simulink model "PV_MG_DroopMPPTV4_TwoFarms"  (R2015a)
settings: Solver=ode3  StartTime=0.0  StopTime=inf  FixedStep=5e-5  RelTol=1e-3
undefined symbols (not defined in the file): Ion, Lithium
libraries: powerlib x61, powerlib_meascontrol x12, simulink x10, fuzblock x3, simulink_extras x3, re_lib x2, electricdrivelib x1
(part 1 of 2)
settings Model: PauseTimes=1.45  CovModelRefEnable=off  Creator=Nady  LastModifiedBy=Nady
settings DataIOCC: SaveFormat=StructureWithTime
settings HardwareCC: ProdBitPerPointer=64  ProdLargestAtomicFloat=Float  ProdIntDivRoundTo=Zero  ProdEndianess=LittleEndian  ProdHWDeviceType=Specified
settings GRTTargetCC: GeneratePreprocessorConditionals=Use local settings

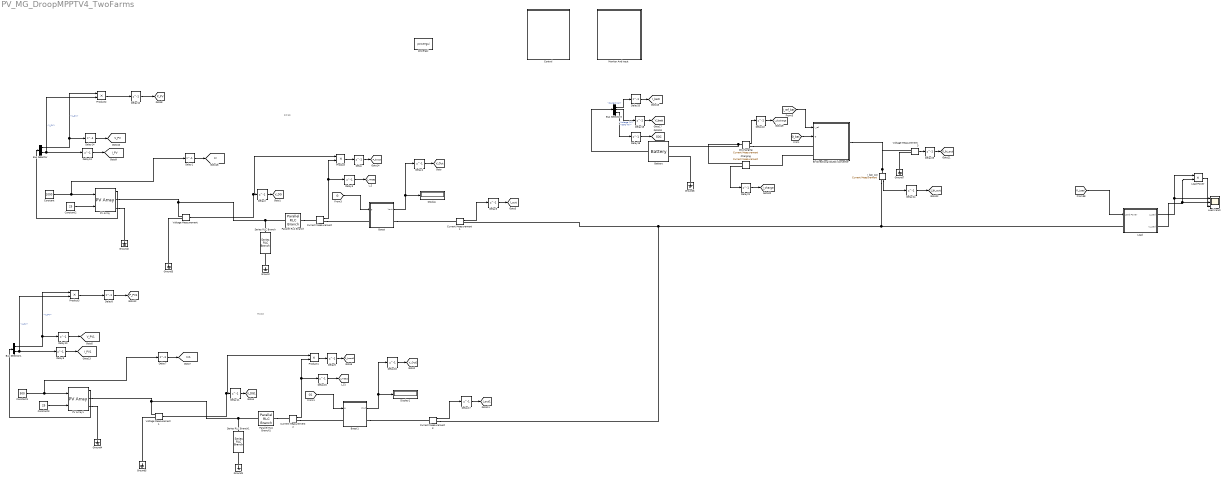
== system PV_MG_DroopMPPTV4_TwoFarms ==
  note: R=10
  note: R=10
  Battery : electricdrivelib/Extra Sources/Battery  BatType=Lithium-Ion  ShowTempParam=off  ThermalPreset=no  NomV=30  NomQ=5.4  SOC=100  Batt_Tr=15  PresetModel=on  MaxQ=5.4  FullV=34.9196  Dis_rate=2.3478  R=0.055556  Normal_OP=4.8835  expZone="[32.4116     0.265304]"  current=[6.5 13 32.5]  Units=Time  Tci=20  NomT=20  T2=-30  MaxQ2=4.8  FullV2=7.1  Normal_OP2=5.72  expZone2="[6.58  1]"  Rca=0.6  ti=1000
  Bi-Directional DC/DC Converter : Subsystem
  Boost : Subsystem
  Boost1 : Subsystem
  Bus Selector : BusSelector  OutputSignals=V_PV,I_PV
  Bus Selector1 : BusSelector  OutputSignals=V_PV,I_PV
  Bus Selector3 : BusSelector  OutputSignals=Current (A),Voltage (V),SOC (%)
  Charging : powerlib/Measurements/Current Measurement  PhasorSimulation=off  OutputType=Complex  PSBequivalent=0
  Constant : Constant  Value=1000
  Constant1 : Constant  Value=500
  Constant2 : Constant  Value=25
  Constant3 : Constant  Value=25
  "Control " : Subsystem
  Current Measurement{,1..3} (4 alike) : powerlib/Measurements/Current Measurement  PhasorSimulation=off  OutputType=Complex  PSBequivalent=0
  Delay{,1..24} (25 alike) : Delay  DelayLength=1  InitialCondition=0
  Discharging : powerlib/Measurements/Current Measurement  PhasorSimulation=off  OutputType=Complex  PSBequivalent=0
  Display : Display
  Display1 : Display
  Ground{,1..7} (8 alike) : powerlib/Elements/Ground  LConnTagsString=a
  I_bat_out : powerlib/Measurements/Current Measurement  PhasorSimulation=off  OutputType=Complex  PSBequivalent=0
  Load : Subsystem
  Load Power : Product
  Load Vand I : Scope  NumInputPorts=3
      settings: TimeRange=auto  MaxDataPoints=5000  SaveToWorkspace=off  SaveName=ScopeData2  YMin=-350.25555~2.15805~-1449.82848  YMax=3150.38643~330.92882~4956.57534  SampleTime=-1
  Monitor And Input : Subsystem
  PV Array : re_lib/Solar/PV Array  Npar=5  Nser=1  PlotType=one module @ 25 deg.C & specified irradiances  S_vec="[ 1000  800 ]"  Temp_C_vec=[35]  ModuleName=Sun Earth Solar Power TDB125x125-36-P 80W  PlotWhenSelected=off  Pm=80.004  Ncell=36  Voc=21.9  Isc=5  Vm=17.7  Im=4.52  beta_Voc_pc=-0.32  alpha_Isc_pc=0.04  beta_Voc=-0.07008  alpha_Isc=0.002  IL=5.0238  I0=3.6974e-11  nI=0.92596  Rsh=70.2892  Rs=0.35567  BAL=off  Tc=1e-6  Tfilter=5e-5
  PV Array1 : re_lib/Solar/PV Array  Npar=5  Nser=1  PlotType=one module @ 25 deg.C & specified irradiances  S_vec="[ 1000  800 ]"  Temp_C_vec=[35]  ModuleName=Sun Earth Solar Power TDB125x125-36-P 80W  PlotWhenSelected=off  Pm=80.004  Ncell=36  Voc=21.9  Isc=5  Vm=17.7  Im=4.52  beta_Voc_pc=-0.32  alpha_Isc_pc=0.04  beta_Voc=-0.07008  alpha_Isc=0.002  IL=5.0238  I0=3.6974e-11  nI=0.92596  Rsh=70.2892  Rs=0.35567  BAL=off  Tc=1e-6  Tfilter=5e-5
  Parallel RLC Branch : powerlib/Elements/Parallel RLC Branch  LConnTagsString=a  RConnTagsString=__new0  BranchType=RL  Resistance=10  Inductance=0.0164  SetiL0=off  InitialCurrent=0  Capacitance=1e-6  Setx0=off  InitialVoltage=0  Measurements=None
  Parallel RLC Branch1 : powerlib/Elements/Parallel RLC Branch  LConnTagsString=a  RConnTagsString=__new0  BranchType=RL  Resistance=10  Inductance=0.0164  SetiL0=off  InitialCurrent=0  Capacitance=1e-6  Setx0=off  InitialVoltage=0  Measurements=None
  Product{,1..3} (4 alike) : Product
  Series RLC Branch : powerlib/Elements/Series RLC Branch  LConnTagsString=__new0  RConnTagsString=__new0  BranchType=C  Resistance=0.1  Inductance=1e-3  SetiL0=off  InitialCurrent=0  Capacitance=0.1  Setx0=off  InitialVoltage=0  Measurements=None
  Series RLC Branch1 : powerlib/Elements/Series RLC Branch  LConnTagsString=__new0  RConnTagsString=__new0  BranchType=C  Resistance=0.1  Inductance=1e-3  SetiL0=off  InitialCurrent=0  Capacitance=0.1  Setx0=off  InitialVoltage=0  Measurements=None
  Voltage Measurement : powerlib/Measurements/Voltage Measurement  PhasorSimulation=off  OutputType=Complex  PSBequivalent=0
  Voltage Measurement1 : powerlib/Measurements/Voltage Measurement  PhasorSimulation=off  OutputType=Complex  PSBequivalent=0
  Voltage Measurement3 : powerlib/Measurements/Voltage Measurement  PhasorSimulation=off  OutputType=Complex  PSBequivalent=0
  powergui : powerlib/powergui  Priority=1  SimulationMode=Discrete  SolverType=Tustin  SampleTime=5e-5  frequency=60  SPID=off  DisableSnubberDevices=off  DisableRonSwitches=off  DisableVfSwitches=off  SwTol=0  DisplayEquations=off  Interpol=off  ExternalGateDelay=off  methode=on  Ts=20  FunctionMessages=off  echomessages=off  HookPort=off  EnableUseOfTLC=off  x0status=blocks  frequencyindice=0  Pbase=100e6  ErrMax=1e-4  Iterations=50  UnitsV=kV  UnitsW=MW  buscounter=0  RestoreLinks=warning  ResistiveCurrentMeasurement=off  Frange=[0:2:500]  Ylog=off  Xlog=on  ShowGrid=off  save=off  variable=ZData  structure=0  ZoomFFT=off  StartTime=0.0  cycles=1  DisplayStyle=1  fundamental=60  FreqAxis=off  MaxFrequency=1000  frequencyindicesteady=1  RmsSteady=1  display=off
  tag scope: I_PV1=global, I_PV=global, I_batt=global, I_bi_out=global, I_charge=global, I_discharge=global, I_meas1=global, I_meas=global, I_out1=global, I_out=global, Irr1=global, Irr=global, P_PV1=global, P_PV=global, P_boost1=global, P_boost=global, SOC=global, V_DG1=global, V_DG=global, V_Out1=global, V_Out=global, V_PV1=global, V_PV=global, V_batt=global, V_bi_out=global
  wires:
  Boost/1(Vout) -> Display/1, Delay4/1
  Voltage Measurement/1 -> Delay2/1, Product/1
  Current Measurement/1 -> Product/2, Delay3/1
  [P_Load] -> Load/1(Load Power)
  Load/1(I_Load) -> Load Power/1, Load Vand I/1
  Load/2(V_Load) -> Load Power/2, Load Vand I/2
  Load Power/1 -> Load Vand I/3
  Current Measurement1/1 -> Delay5/1
  Product/1 -> Delay/1
  Delay/1 -> [P_boost]
  Delay1/1 -> [Irr]
  Delay2/1 -> [V_DG]
  Delay3/1 -> [I_meas]
  Delay4/1 -> [V_Out]
  Delay5/1 -> [I_out]
  Constant2/1 -> PV Array/2
  Bus Selector/1 -> Delay14/1, Product2/1  "<V_PV>"
  Bus Selector/2 -> Delay13/1, Product2/2  "<I_PV>"
  PV Array/1 -> Bus Selector/1
  Constant/1 -> PV Array/1, Delay1/1
  Product2/1 -> Delay12/1
  Delay12/1 -> [P_PV]
  [G] -> Boost/1(g)
  Delay13/1 -> [I_PV]
  Delay14/1 -> [V_PV]
  Boost1/1(Vout) -> Delay16/1, Display1/1
  Voltage Measurement1/1 -> Product1/1, Delay11/1
  Current Measurement2/1 -> Delay15/1, Product1/2
  Current Measurement3/1 -> Delay17/1
  Product1/1 -> Delay6/1
  Delay6/1 -> [P_boost1]
  Delay7/1 -> [Irr1]
  Delay11/1 -> [V_DG1]
  Delay15/1 -> [I_meas1]
  Delay16/1 -> [V_Out1]
  Delay17/1 -> [I_out1]
  Constant3/1 -> PV Array1/2
  Bus Selector1/1 -> Product3/1, Delay10/1  "<V_PV>"
  Bus Selector1/2 -> Product3/2, Delay9/1  "<I_PV>"
  PV Array1/1 -> Bus Selector1/1
  Constant1/1 -> Delay7/1, PV Array1/1
  Product3/1 -> Delay8/1
  Delay8/1 -> [P_PV1]
  [G1] -> Boost1/1(g)
  Delay9/1 -> [I_PV1]
  Delay10/1 -> [V_PV1]
  Discharging/1 -> Delay22/1
  Charging/1 -> Delay21/1
  [G_bat] -> Bi-Directional DC/DC Converter/2(G)
  Voltage Measurement3/1 -> Delay23/1
  I_bat_out/1 -> Delay24/1
  Battery/1 -> Bus Selector3/1
  Bus Selector3/1 -> Delay20/1  "<Current (A)>"
  Bus Selector3/2 -> Delay18/1  "<Voltage (V)>"
  [I_ref_bat] -> Bi-Directional DC/DC Converter/1(I_ref)
  Bus Selector3/3 -> Delay19/1  "<SOC (%)>"
  Delay19/1 -> [SOC]
  Delay18/1 -> [V_batt]
  Delay20/1 -> [I_batt]
  Delay21/1 -> [I_charge]
  Delay22/1 -> [I_discharge]
  Delay24/1 -> [I_bi_out]
  Delay23/1 -> [V_bi_out]
  connections:
  Current Measurement/RConn1 -- Boost/LConn1
  Voltage Measurement/LConn1 -- PV Array/RConn1 -- Parallel RLC Branch/LConn1 -- Series RLC Branch/LConn1
  Boost/RConn1 -- Current Measurement1/LConn1
  Load/LConn1 -- I_bat_out/RConn1 -- Current Measurement3/RConn1 -- Current Measurement1/RConn1
  Ground/LConn1 -- Series RLC Branch/RConn1
  PV Array/RConn2 -- Ground2/LConn1
  Voltage Measurement/LConn2 -- Ground3/LConn1
  Parallel RLC Branch/RConn1 -- Current Measurement/LConn1
  PV Array1/RConn1 -- Series RLC Branch1/LConn1 -- Parallel RLC Branch1/LConn1 -- Voltage Measurement1/LConn1
  Parallel RLC Branch1/RConn1 -- Current Measurement2/LConn1
  PV Array1/RConn2 -- Ground4/LConn1
  Voltage Measurement1/LConn2 -- Ground5/LConn1
  Current Measurement2/RConn1 -- Boost1/LConn1
  Ground1/LConn1 -- Series RLC Branch1/RConn1
  Boost1/RConn1 -- Current Measurement3/LConn1
  I_bat_out/LConn1 -- Bi-Directional DC/DC Converter/RConn1 -- Voltage Measurement3/LConn1
  Discharging/LConn1 -- Battery/LConn1 -- Charging/RConn1
  Ground7/LConn1 -- Voltage Measurement3/LConn2
  Ground6/LConn1 -- Battery/LConn2
  Discharging/RConn1 -- Bi-Directional DC/DC Converter/LConn1
  Bi-Directional DC/DC Converter/LConn2 -- Charging/LConn1

== system PV_MG_DroopMPPTV4_TwoFarms/Bi-Directional DC//DC Converter ==
  I_ref : Inport
  G : Inport  Port=2
  Boost : Subsystem
  Buck : Subsystem
  Constant2 : Constant  Value=0
  Constant3 : Constant  Value=0
  G1 : InportShadow  Port=2
  I_ref1 : InportShadow
  Switch1 : Switch  Criteria=u2 > Threshold
  Switch2 : Switch  Criteria=u2 > Threshold
  Boost_In : PMIOPort  Port=1  Side=Left
  V_Bus : PMIOPort  Port=2  Side=Right
  Buck_out : PMIOPort  Port=3  Side=Left
  wires:
  I_ref/1 -> Switch2/2
  Switch1/1 -> Buck/1(G)
  G/1 -> Switch1/3
  Switch2/1 -> Boost/1(g)
  G1/1 -> Switch2/1
  Constant2/1 -> Switch1/1
  Constant3/1 -> Switch2/3
  I_ref1/1 -> Switch1/2
  connections:
  Buck_out/RConn1 -- Buck/LConn1
  Boost_In/RConn1 -- Boost/LConn1
  Boost/RConn1 -- Buck/RConn1 -- V_Bus/RConn1

== system PV_MG_DroopMPPTV4_TwoFarms/Boost ==
  g : Inport
  C_LP : powerlib/Elements/Series RLC Branch  LConnTagsString=__new0  RConnTagsString=__new0  BranchType=R  Resistance=1  Inductance=1e-3  SetiL0=off  InitialCurrent=0  Capacitance=0.004  Setx0=off  InitialVoltage=0  Measurements=None
  Data Type Conversion : DataTypeConversion  OutDataTypeStr=boolean
  Ground : powerlib/Elements/Ground  LConnTagsString=a
  IGBT : powerlib/Power Electronics/IGBT  Ron=0.001  Lon=0  Vf=1  Tf=1e-6  Tt=2e-6  IC=0  Rs=1e5  Cs=inf  Measurements=on
  IGBT1 : powerlib/Power Electronics/IGBT  Ron=0.001  Lon=0  Vf=1  Tf=1e-6  Tt=2e-6  IC=0  Rs=1e5  Cs=inf  Measurements=on
  L_LP : powerlib/Elements/Series RLC Branch  LConnTagsString=__new0  RConnTagsString=__new0  BranchType=L  Resistance=0.01  Inductance=0.0164  SetiL0=off  InitialCurrent=0  Capacitance=6e-2  Setx0=off  InitialVoltage=0  Measurements=None
  Logical Operator : Logic  Operator=NOT  AllPortsSameDT=off  OutDataTypeStr=boolean
  R_LP1 : powerlib/Elements/Series RLC Branch  LConnTagsString=__new0  RConnTagsString=__new0  BranchType=L  Resistance=0.01  Inductance=7e-3  SetiL0=off  InitialCurrent=0  Capacitance=6e-2  Setx0=off  InitialVoltage=0  Measurements=None
  Series RLC Branch3 : powerlib/Elements/Series RLC Branch  LConnTagsString=__new0  RConnTagsString=__new0  BranchType=C  Resistance=0.005  Inductance=1e-3  SetiL0=off  InitialCurrent=0  Capacitance=6e-3  Setx0=off  InitialVoltage=0  Measurements=None
  Voltage Measurement : powerlib/Measurements/Voltage Measurement  PhasorSimulation=off  OutputType=Complex  PSBequivalent=0
  Vin (Il) : PMIOPort  Tag=PMCPort  Port=1  Side=Left
  Vc : PMIOPort  Tag=PMCPort  Port=2  Side=Right
  Vout : Outport
  wires:
  Voltage Measurement/1 -> Vout/1
  g/1 -> Data Type Conversion/1, IGBT/1
  Data Type Conversion/1 -> Logical Operator/1
  Logical Operator/1 -> IGBT1/1
  connections:
  IGBT/RConn1 -- Ground/LConn1 -- Voltage Measurement/LConn2 -- Series RLC Branch3/RConn1
  IGBT1/LConn1 -- R_LP1/LConn1 -- IGBT/LConn1
  R_LP1/RConn1 -- Vin (Il)/RConn1
  Vc/RConn1 -- C_LP/LConn1 -- L_LP/LConn1 -- Voltage Measurement/LConn1
  Series RLC Branch3/LConn1 -- C_LP/RConn1 -- L_LP/RConn1 -- IGBT1/RConn1

== system PV_MG_DroopMPPTV4_TwoFarms/Boost1 ==
  g : Inport
  C_LP : powerlib/Elements/Series RLC Branch  LConnTagsString=__new0  RConnTagsString=__new0  BranchType=R  Resistance=1  Inductance=1e-3  SetiL0=off  InitialCurrent=0  Capacitance=0.004  Setx0=off  InitialVoltage=0  Measurements=None
  Data Type Conversion : DataTypeConversion  OutDataTypeStr=boolean
  Ground : powerlib/Elements/Ground  LConnTagsString=a
  IGBT : powerlib/Power Electronics/IGBT  Ron=0.001  Lon=0  Vf=1  Tf=1e-6  Tt=2e-6  IC=0  Rs=1e5  Cs=inf  Measurements=on
  IGBT1 : powerlib/Power Electronics/IGBT  Ron=0.001  Lon=0  Vf=1  Tf=1e-6  Tt=2e-6  IC=0  Rs=1e5  Cs=inf  Measurements=on
  L_LP : powerlib/Elements/Series RLC Branch  LConnTagsString=__new0  RConnTagsString=__new0  BranchType=L  Resistance=0.01  Inductance=0.0164  SetiL0=off  InitialCurrent=0  Capacitance=6e-2  Setx0=off  InitialVoltage=0  Measurements=None
  Logical Operator : Logic  Operator=NOT  AllPortsSameDT=off  OutDataTypeStr=boolean
  R_LP1 : powerlib/Elements/Series RLC Branch  LConnTagsString=__new0  RConnTagsString=__new0  BranchType=L  Resistance=0.01  Inductance=7e-3  SetiL0=off  InitialCurrent=0  Capacitance=6e-2  Setx0=off  InitialVoltage=0  Measurements=None
  Series RLC Branch3 : powerlib/Elements/Series RLC Branch  LConnTagsString=__new0  RConnTagsString=__new0  BranchType=C  Resistance=0.005  Inductance=1e-3  SetiL0=off  InitialCurrent=0  Capacitance=6e-3  Setx0=off  InitialVoltage=0  Measurements=None
  Voltage Measurement : powerlib/Measurements/Voltage Measurement  PhasorSimulation=off  OutputType=Complex  PSBequivalent=0
  Vin (Il) : PMIOPort  Tag=PMCPort  Port=1  Side=Left
  Vc : PMIOPort  Tag=PMCPort  Port=2  Side=Right
  Vout : Outport
  wires:
  Logical Operator/1 -> IGBT1/1
  Data Type Conversion/1 -> Logical Operator/1
  g/1 -> IGBT/1, Data Type Conversion/1
  Voltage Measurement/1 -> Vout/1
  connections:
  IGBT1/RConn1 -- Series RLC Branch3/LConn1 -- L_LP/RConn1 -- C_LP/RConn1
  Voltage Measurement/LConn1 -- C_LP/LConn1 -- L_LP/LConn1 -- Vc/RConn1
  R_LP1/RConn1 -- Vin (Il)/RConn1
  IGBT/LConn1 -- R_LP1/LConn1 -- IGBT1/LConn1
  Series RLC Branch3/RConn1 -- Voltage Measurement/LConn2 -- Ground/LConn1 -- IGBT/RConn1

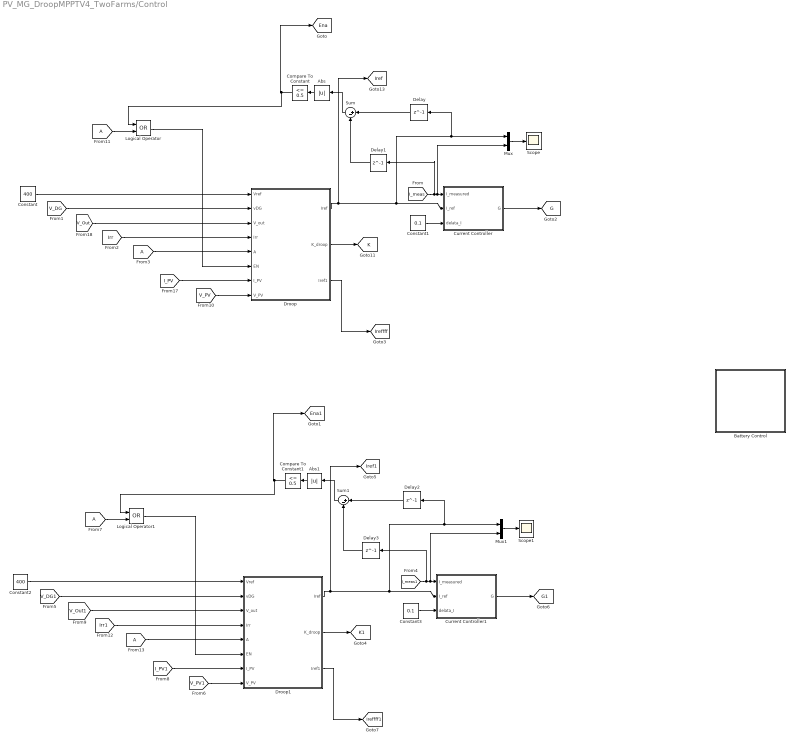
== system PV_MG_DroopMPPTV4_TwoFarms/Control  ==
  Abs : Abs
  Abs1 : Abs
  Battery Control : Subsystem
  Compare To Constant : simulink/Logic and Bit Operations/Compare To Constant  relop=<=  const=0.5  OutDataTypeStr=boolean
  Compare To Constant1 : simulink/Logic and Bit Operations/Compare To Constant  relop=<=  const=0.5  OutDataTypeStr=boolean
  Constant : Constant  Value=400  SampleTime=5e-5
  Constant1 : Constant  Value=0.1  SampleTime=0
  Constant2 : Constant  Value=400  SampleTime=5e-5
  Constant3 : Constant  Value=0.1  SampleTime=0
  Current Controller : Subsystem  TreatAsAtomicUnit=on
  Current Controller1 : Subsystem  TreatAsAtomicUnit=on
  Delay{,1..3} (4 alike) : Delay  DelayLength=1  InitialCondition=0
  Droop : Subsystem  TreatAsAtomicUnit=on
  Droop1 : Subsystem  TreatAsAtomicUnit=on
  Logical Operator : Logic  Operator=OR  AllPortsSameDT=off  OutDataTypeStr=boolean
  Logical Operator1 : Logic  Operator=OR  AllPortsSameDT=off  OutDataTypeStr=boolean
  Mux : Mux  Inputs=2
  Mux1 : Mux  Inputs=2
  Scope : Scope
      settings: TimeRange=auto  MaxDataPoints=5000  SaveToWorkspace=off  SaveName=ScopeData4  YMin=-2.92442  YMax=26.28218  SampleTime=-1
  Scope1 : Scope
      settings: TimeRange=auto  LimitDataPoints=on  MaxDataPoints=5000  SaveToWorkspace=off  YMin=-10  YMax=10  SampleTime=-1  DataFormat=Array
  Sum : Sum  Inputs=|+-
  Sum1 : Sum  Inputs=|+-
  tag scope: Ena1=global, Ena=global, G1=global, G=global, Iref1=global, Iref=global, Ireffff1=global, Ireffff=global, K1=global, K=global
  wires:
  Droop/1(Iref) -> Current Controller/2(I_ref), Delay/1, Mux/1, [Iref]
  Constant/1 -> Droop/1(Vref)
  [I_meas] -> Delay1/1, Mux/2, Current Controller/1(I_measured)
  Constant1/1 -> Current Controller/3(delata_I)
  Current Controller/1(G) -> [G]
  Droop/2(K_droop) -> [K]
  Mux/1 -> Scope/1
  Droop/3(Iref1) -> [Ireffff]
  Sum/1 -> Abs/1
  Abs/1 -> Compare To Constant/1
  Compare To Constant/1 -> Logical Operator/1, [Ena]
  Delay/1 -> Sum/1
  Delay1/1 -> Sum/2
  [V_DG] -> Droop/2(vDG)
  [V_Out] -> Droop/3(V_out)
  [Irr] -> Droop/4(Irr)
  [A] -> Droop/5(A)
  [I_PV] -> Droop/7(I_PV)
  [V_PV] -> Droop/8(V_PV)
  [A] -> Logical Operator/2
  Logical Operator/1 -> Droop/6(EN)
  Droop1/1(Iref) -> [Iref1], Mux1/1, Delay2/1, Current Controller1/2(I_ref)
  Constant2/1 -> Droop1/1(Vref)
  [I_meas1] -> Current Controller1/1(I_measured), Mux1/2, Delay3/1
  Constant3/1 -> Current Controller1/3(delata_I)
  Current Controller1/1(G) -> [G1]
  Droop1/2(K_droop) -> [K1]
  Mux1/1 -> Scope1/1
  Droop1/3(Iref1) -> [Ireffff1]
  Sum1/1 -> Abs1/1
  Abs1/1 -> Compare To Constant1/1
  Compare To Constant1/1 -> [Ena1], Logical Operator1/1
  Delay2/1 -> Sum1/1
  Delay3/1 -> Sum1/2
  [V_DG1] -> Droop1/2(vDG)
  [V_Out1] -> Droop1/3(V_out)
  [Irr1] -> Droop1/4(Irr)
  [A] -> Droop1/5(A)
  [I_PV1] -> Droop1/7(I_PV)
  [V_PV1] -> Droop1/8(V_PV)
  [A] -> Logical Operator1/2
  Logical Operator1/1 -> Droop1/6(EN)

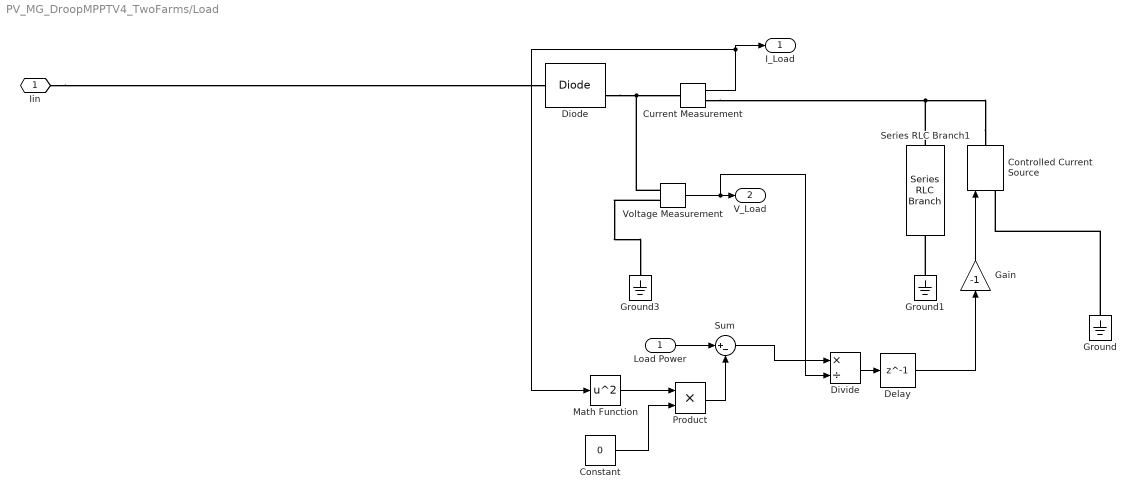
== system PV_MG_DroopMPPTV4_TwoFarms/Load ==
  Load Power : Inport
  Constant : Constant  Value=0
  Controlled Current Source : powerlib/Electrical Sources/Controlled Current Source  Initialize=on  Source_Type=AC  Amplitude=0  Phase=0  Frequency=0  Measurements=None
  Current Measurement : powerlib/Measurements/Current Measurement  PhasorSimulation=off  OutputType=Complex  PSBequivalent=0
  Delay : Delay  DelayLength=1  InitialCondition=0
  Diode : powerlib/Power Electronics/Diode  Ron=0.001  Lon=0  Vf=0.8  IC=0  UseSnubber=off  Rs=500  Cs=250e-9  Measurements=on
  Divide : Product  Inputs=*/
  Gain : Gain  Gain=-1
  Ground : powerlib/Elements/Ground  LConnTagsString=a
  Ground1 : powerlib/Elements/Ground  LConnTagsString=a
  Ground3 : powerlib/Elements/Ground  LConnTagsString=a
  Math Function : Math  Operator=square  SaturateOnIntegerOverflow=on
  Product : Product
  Series RLC Branch1 : powerlib/Elements/Series RLC Branch  LConnTagsString=__new0  RConnTagsString=__new0  BranchType=C  Resistance=1  Inductance=1e-3  SetiL0=off  InitialCurrent=0  Capacitance=1e-3  Setx0=off  InitialVoltage=0  Measurements=None
  Sum : Sum  Inputs=|+-
  Voltage Measurement : powerlib/Measurements/Voltage Measurement  PhasorSimulation=off  OutputType=Complex  PSBequivalent=0
  Iin : PMIOPort  Port=1  Side=Left
  I_Load : Outport
  V_Load : Outport  Port=2
  wires:
  Gain/1 -> Controlled Current Source/1
  Divide/1 -> Delay/1
  Delay/1 -> Gain/1
  Math Function/1 -> Product/1
  Constant/1 -> Product/2
  Load Power/1 -> Sum/1
  Product/1 -> Sum/2
  Sum/1 -> Divide/1
  Current Measurement/1 -> Math Function/1, I_Load/1
  Voltage Measurement/1 -> Divide/2, V_Load/1
  connections:
  Voltage Measurement/LConn1 -- Diode/RConn1 -- Current Measurement/LConn1
  Voltage Measurement/LConn2 -- Ground3/LConn1
  Ground/LConn1 -- Controlled Current Source/LConn1
  Controlled Current Source/RConn1 -- Current Measurement/RConn1 -- Series RLC Branch1/LConn1
  Ground1/LConn1 -- Series RLC Branch1/RConn1
  Iin/RConn1 -- Diode/LConn1

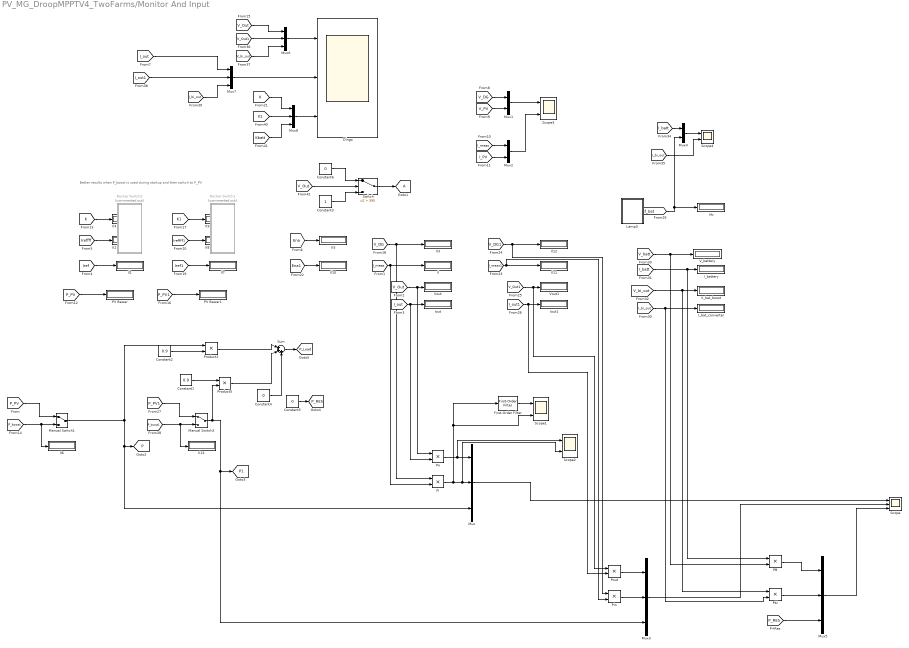
== system PV_MG_DroopMPPTV4_TwoFarms/Monitor And Input ==
  note: Better results when P_boost is used during startup and then switch to P_PV
  Constant1 : Constant  Value=0.9  SampleTime=0
  Constant2 : Constant  Value=0.9  SampleTime=0
  Constant3 : Constant  SampleTime=0
  Constant4 : Constant  Value=0  SampleTime=0
  Constant5 : Constant  Value=0  SampleTime=0
  Constant6 : Constant  Value=0  SampleTime=0
  Dingo : Scope  NumInputPorts=3
      settings: TimeRange=3.8087  ShowLegends=on  MaxDataPoints=5000  SaveToWorkspace=off  YMin=-51.0886~-5.15693~-0.5  YMax=453.41004~10.3251~4.5  SampleTime=-1
  First-Order Filter : powerlib_meascontrol/Filters/First-Order Filter  FilterType=Lowpass  Tc=1/400  Ts=5e-5  Initialize=off  Vac_Init=[0, 0, 60]  Vdc_Init=0  PlotResponse=off  FreqRange="[0,  200,  1]"
  I_bat_converter : Display
  I_battery : Display
  Il{,1..13} (14 alike) : Display
  Iout : Display
  Iout1 : Display
  Irb : Display
  Lamp3 : Subsystem  DialogController=hmiCreateDDGDialog  mask(MWDashboardBlock){webBlockId=a411fb8a-8cc9-40be-9d83-47cf8fd6e8c1, webBlockType=lamp, ShowInLibBrowser=on, ShowInitialText=on, HMISrcModelName=[]}
      mask prompts: webBlockType "WebBlock Type"; HMISrcModelName "Source Model"
      mask Help: helpview([docroot '/mapfiles/simulink.map'], 'hmi_lamp')
      mask Display:
      | if strcmp(get_param(bdroot(gcb),'BlockDiagramType'), 'library')
      |     image([(matlabroot) '/toolbox/simulink/hmi/icons/Lamp.png']);
      | end
  Manual Switch1 : ManualSwitch
  Manual Switch2 : ManualSwitch
  Mux{,3,5..8} (6 alike) : Mux  Inputs=3
  Mux1 : Mux  Inputs=2
  Mux2 : Mux  Inputs=2
  Mux4 : Mux  Inputs=2
  PB : Product
  PV Bawar : Display
  PV Bawar1 : Display
  Pbi : Product
  Pi : Product
  Pin : Product
  Po : Product
  Pout : Product
  Product1 : Product
  Product5 : Product
  Rocker Switch1 : Subsystem  Commented=on  DialogController=hmiCreateDDGDialog  mask(MWDashboardBlock){webBlockId=5e99b1b3-df07-4cef-a3f6-0ddfeeb3b4e9, webBlockType=rockerswitch, ShowInLibBrowser=on, ShowInitialText=on, HMISrcModelName=[]}
      mask prompts: webBlockId "WebBlock Id"; webBlockType "WebBlock Type"; HMISrcModelName "Source Model"
      mask Help: helpview([docroot '/mapfiles/simulink.map'], 'hmi_rocker_switch')
      mask Display:
      | if strcmp(get_param(bdroot(gcb),'BlockDiagramType'), 'library')
      |     image([(matlabroot) '/toolbox/simulink/hmi/icons/RockerSwitch.png']);
      | end
  Rocker Switch2 : Subsystem  Commented=on  DialogController=hmiCreateDDGDialog  mask(MWDashboardBlock){webBlockId=5e99b1b3-df07-4cef-a3f6-0ddfeeb3b4e9, webBlockType=rockerswitch, ShowInLibBrowser=on, ShowInitialText=on, HMISrcModelName=[]}
      mask prompts: webBlockId "WebBlock Id"; webBlockType "WebBlock Type"; HMISrcModelName "Source Model"
      mask Help: helpview([docroot '/mapfiles/simulink.map'], 'hmi_rocker_switch')
      mask Display:
      | if strcmp(get_param(bdroot(gcb),'BlockDiagramType'), 'library')
      |     image([(matlabroot) '/toolbox/simulink/hmi/icons/RockerSwitch.png']);
      | end
  Scope : Scope  NumInputPorts=3
      settings: TimeRange=auto  ShowLegends=on  MaxDataPoints=5000  SaveToWorkspace=off  YMin=-1455.53207~-18.55249~-8367.82947  YMax=5487.64172~87.00582~3974.25451  SampleTime=-1
  Scope{1..4} (4 alike) : Scope  NumInputPorts=2
      Scope1 settings: TimeRange=auto  MaxDataPoints=5000  SaveToWorkspace=off  SaveName=ScopeData  YMin=-102.309~-5  YMax=495.80827~5  SampleTime=-1
      Scope2 settings: TimeRange=auto  MaxDataPoints=5000  SaveToWorkspace=off  SaveName=ScopeData2  YMin=-909447.34641~-488.47375  YMax=104856.12265~844.68145  SampleTime=-1
      Scope3 settings: TimeRange=auto  MaxDataPoints=5000  SaveToWorkspace=off  SaveName=ScopeData3  YMin=-2.6975~-3.12322  YMax=24.27751~28.10897  SampleTime=-1
      Scope4 settings: TimeRange=auto  MaxDataPoints=5000  SaveToWorkspace=off  SaveName=ScopeData6  YMin=-100~-60  YMax=500~120  SampleTime=-1
  Sum : Sum  Inputs=|+++
  Switch : Switch  Criteria=u2 > Threshold  Threshold=395
  V_bat_boost : Display
  V_battery : Display
  Vout : Display
  Vout1 : Display
  tag scope: A=global, P1=global, P=global, P_Load=global, P_RES=global
  wires:
  [I_meas] -> Pi/2, Il/1
  [V_Out] -> Po/1, Vout/1
  [I_out] -> Po/2, Iout/1
  [V_DG] -> Il3/1, Pi/1
  Po/1 -> Scope2/1, Mux/1
  Pi/1 -> First-Order Filter/1, Scope1/2, Scope2/2, Mux/2
  [P_boost] -> Manual Switch1/2, Il6/1
  [P_PV] -> Manual Switch1/1
  [Iref] -> Il1/1
  [Ireffff] -> Il2/1
  Manual Switch1/1 -> Product1/1, [P], Mux/3
  Constant2/1 -> Product1/2
  [Ena] -> Il5/1
  First-Order Filter/1 -> Scope1/1
  Mux1/1 -> Scope3/1
  [V_DG] -> Mux1/1
  [V_PV] -> Mux1/2
  Mux2/1 -> Scope3/2
  [I_meas] -> Mux2/1
  [I_PV] -> Mux2/2
  [P_PV] -> PV Bawar/1
  [K] -> Il4/1
  [Iref1] -> Il7/1
  [Ireffff1] -> Il8/1
  [P_PV1] -> PV Bawar1/1
  [K1] -> Il9/1
  [Ena1] -> Il10/1
  [I_meas1] -> Pin/2, Il11/1
  [V_Out1] -> Pout/1, Vout1/1
  [I_out1] -> Pout/2, Iout1/1
  [V_DG1] -> Pin/1, Il12/1
  Pout/1 -> Mux3/1
  Pin/1 -> Mux3/2
  [P_boost1] -> Il13/1, Manual Switch2/2
  [P_PV1] -> Manual Switch2/1
  Manual Switch2/1 -> [P1], Mux3/3, Product5/2
  Product1/1 -> Sum/1
  Constant1/1 -> Product5/1
  Product5/1 -> Sum/2
  Sum/1 -> [P_Load]
  Constant4/1 -> Sum/3
  [I_ref_bat] -> Irb/1, Mux4/2
  [I_batt] -> PB/1, I_battery/1
  [V_bi_out] -> Pbi/1, V_bat_boost/1
  [I_bi_out] -> Pbi/2, I_bat_converter/1
  [V_batt] -> PB/2, V_battery/1
  [I_batt] -> Mux4/1
  Mux4/1 -> Scope4/1
  [I_bi_out] -> Scope4/2
  Constant5/1 -> [P_RES]
  Mux/1 -> Scope/1
  Mux3/1 -> Scope/2
  PB/1 -> Mux5/1
  Pbi/1 -> Mux5/2
  [P_RES] -> Mux5/3
  Mux5/1 -> Scope/3
  [V_Out] -> Mux6/1
  [V_Out1] -> Mux6/2
  [V_bi_out] -> Mux6/3
  [I_out1] -> Mux7/2
  [I_out] -> Mux7/1
  [I_bi_out] -> Mux7/3
  Mux6/1 -> Dingo/1
  Mux7/1 -> Dingo/2
  [K1] -> Mux8/2
  [K] -> Mux8/1
  [Kbatt] -> Mux8/3
  Mux8/1 -> Dingo/3
  Constant3/1 -> Switch/3
  Constant6/1 -> Switch/1
  [V_Out] -> Switch/2
  Switch/1 -> [A]

== system PV_MG_DroopMPPTV4_TwoFarms/Bi-Directional DC//DC Converter/Boost ==
  g : Inport
  C_LP : powerlib/Elements/Series RLC Branch  LConnTagsString=__new0  RConnTagsString=__new0  BranchType=R  Resistance=1  Inductance=1e-3  SetiL0=off  InitialCurrent=0  Capacitance=0.004  Setx0=off  InitialVoltage=0  Measurements=None
  Data Type Conversion : DataTypeConversion  OutDataTypeStr=boolean
  Ground : powerlib/Elements/Ground  LConnTagsString=a
  IGBT : powerlib/Power Electronics/IGBT  Ron=0.001  Lon=0  Vf=1  Tf=1e-6  Tt=2e-6  IC=0  Rs=1e5  Cs=inf  Measurements=on
  IGBT1 : powerlib/Power Electronics/IGBT  Ron=0.001  Lon=0  Vf=1  Tf=1e-6  Tt=2e-6  IC=0  Rs=1e5  Cs=inf  Measurements=on
  L_LP : powerlib/Elements/Series RLC Branch  LConnTagsString=__new0  RConnTagsString=__new0  BranchType=L  Resistance=0.01  Inductance=0.0164  SetiL0=off  InitialCurrent=0  Capacitance=6e-2  Setx0=off  InitialVoltage=0  Measurements=None
  Logical Operator : Logic  Operator=NOT  AllPortsSameDT=off  OutDataTypeStr=boolean
  Series RLC Branch1 : powerlib/Elements/Series RLC Branch  LConnTagsString=__new0  RConnTagsString=__new0  BranchType=L  Resistance=0.1  Inductance=7e-3  SetiL0=off  InitialCurrent=0  Capacitance=1e-6  Setx0=off  InitialVoltage=0  Measurements=None
  Series RLC Branch3 : powerlib/Elements/Series RLC Branch  LConnTagsString=__new0  RConnTagsString=__new0  BranchType=C  Resistance=0.1  Inductance=1e-3  SetiL0=off  InitialCurrent=0  Capacitance=6e-2  Setx0=off  InitialVoltage=0  Measurements=None
  Vin (Il) : PMIOPort  Tag=PMCPort  Port=1  Side=Left
  Vc : PMIOPort  Tag=PMCPort  Port=2  Side=Right
  wires:
  g/1 -> Data Type Conversion/1, IGBT/1
  Data Type Conversion/1 -> Logical Operator/1
  Logical Operator/1 -> IGBT1/1
  connections:
  Series RLC Branch3/LConn1 -- C_LP/RConn1 -- L_LP/RConn1 -- IGBT1/RConn1
  IGBT/RConn1 -- Ground/LConn1 -- Series RLC Branch3/RConn1
  IGBT/LConn1 -- IGBT1/LConn1 -- Series RLC Branch1/LConn1
  Vin (Il)/RConn1 -- Series RLC Branch1/RConn1
  L_LP/LConn1 -- C_LP/LConn1 -- Vc/RConn1

== system PV_MG_DroopMPPTV4_TwoFarms/Bi-Directional DC//DC Converter/Buck ==
  G : Inport
  C_LP : powerlib/Elements/Series RLC Branch  LConnTagsString=__new0  RConnTagsString=__new0  BranchType=R  Resistance=10  Inductance=1e-3  SetiL0=off  InitialCurrent=0  Capacitance=0.004  Setx0=off  InitialVoltage=0  Measurements=None
  Cap : powerlib/Elements/Series RLC Branch  LConnTagsString=__new0  RConnTagsString=__new0  BranchType=C  Resistance=0.1  Inductance=1e-3  SetiL0=off  InitialCurrent=0  Capacitance=1e-3  Setx0=off  InitialVoltage=0  Measurements=None
  Diode : powerlib/Power Electronics/Diode  Ron=0.001  Lon=0  Vf=0.8  IC=0  UseSnubber=off  Rs=500  Cs=250e-9  Measurements=on
  Ground1 : powerlib/Elements/Ground  LConnTagsString=a
  IGBT : powerlib/Power Electronics/IGBT  Ron=0.001  Lon=0  Vf=1  Tf=1e-6  Tt=2e-6  IC=0  Rs=1e5  Cs=inf  Measurements=on
  Ind : powerlib/Elements/Series RLC Branch  LConnTagsString=__new0  RConnTagsString=__new0  BranchType=L  Resistance=1  Inductance=9e-3  SetiL0=off  InitialCurrent=0  Capacitance=1e-6  Setx0=off  InitialVoltage=0  Measurements=None
  L_LP : powerlib/Elements/Series RLC Branch  LConnTagsString=__new0  RConnTagsString=__new0  BranchType=L  Resistance=0.01  Inductance=0.0164  SetiL0=off  InitialCurrent=0  Capacitance=6e-2  Setx0=off  InitialVoltage=0  Measurements=None
  VL : PMIOPort  Port=1  Side=Left
  VH : PMIOPort  Port=2  Side=Right
  wires:
  G/1 -> IGBT/1
  connections:
  Diode/LConn1 -- Ground1/LConn1 -- Cap/RConn1
  IGBT/RConn1 -- Diode/RConn1 -- Ind/RConn1
  VL/RConn1 -- Ind/LConn1
  IGBT/LConn1 -- C_LP/RConn1 -- L_LP/RConn1 -- Cap/LConn1
  L_LP/LConn1 -- C_LP/LConn1 -- VH/RConn1

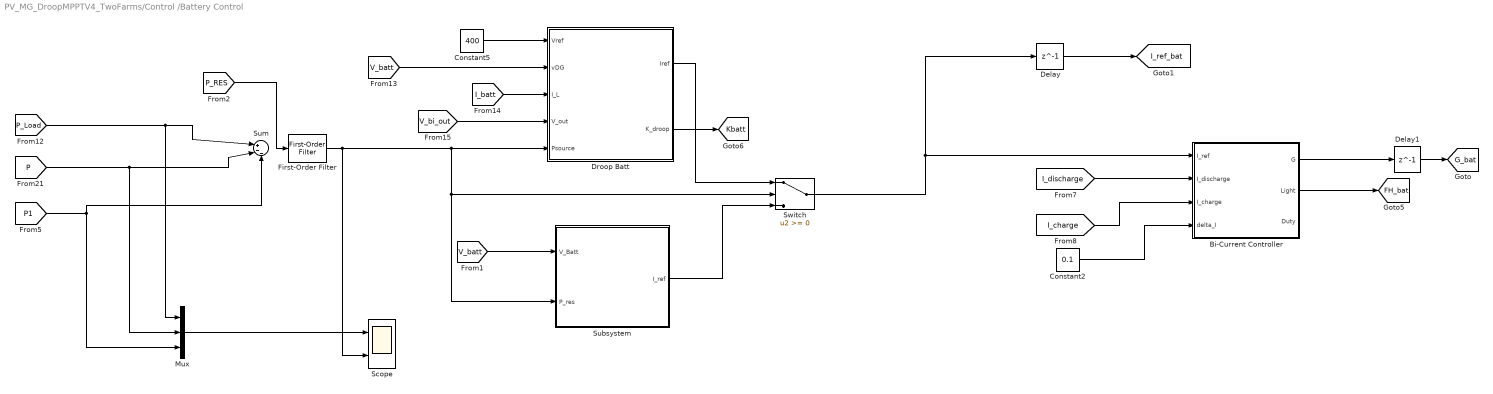
== system PV_MG_DroopMPPTV4_TwoFarms/Control /Battery Control ==
  Bi-Current Controller : Subsystem  TreatAsAtomicUnit=on
  Constant2 : Constant  Value=0.1
  Constant5 : Constant  Value=400  SampleTime=5e-5
  Delay : Delay  DelayLength=1  InitialCondition=0
  Delay1 : Delay  DelayLength=1  InitialCondition=0
  Droop Batt : Subsystem  TreatAsAtomicUnit=on
  First-Order Filter : powerlib_meascontrol/Filters/First-Order Filter  FilterType=Lowpass  Tc=1/400  Ts=0  Initialize=off  Vac_Init=[0, 0, 60]  Vdc_Init=0  PlotResponse=off  FreqRange="[0,  5000,  1]"
  Mux : Mux  Inputs=3
  Scope : Scope  NumInputPorts=2
      settings: TimeRange=auto  MaxDataPoints=5000  SaveToWorkspace=off  SaveName=ScopeData3  YMin=-25~-3e-14  YMax=425~3e-14  SampleTime=-1  DataFormat=Array
  Subsystem : Subsystem
  Sum : Sum  Inputs=|+--
  Switch : Switch
  tag scope: FH_bat=global, G_bat=global, I_ref_bat=global, Kbatt=global
  wires:
  Droop Batt/2(K_droop) -> [Kbatt]
  [I_discharge] -> Bi-Current Controller/2(I_discharge)
  [I_charge] -> Bi-Current Controller/3(I_charge)
  Bi-Current Controller/2(Light) -> [FH_bat]
  Constant2/1 -> Bi-Current Controller/4(delta_I)
  [P] -> Mux/2, Sum/2
  [P_Load] -> Mux/1, Sum/1
  [I_batt] -> Droop Batt/3(I_L)
  [V_batt] -> Droop Batt/2(vDG)
  [V_bi_out] -> Droop Batt/4(V_out)
  Constant5/1 -> Droop Batt/1(Vref)
  [P1] -> Sum/3, Mux/3
  [V_batt] -> Subsystem/1(V_Batt)
  Droop Batt/1(Iref) -> Switch/1
  Subsystem/1(I_ref) -> Switch/3
  Switch/1 -> Delay/1, Bi-Current Controller/1(I_ref)
  Bi-Current Controller/1(G) -> Delay1/1
  Delay/1 -> [I_ref_bat]
  Delay1/1 -> [G_bat]
  Mux/1 -> Scope/1
  First-Order Filter/1 -> Scope/2, Subsystem/2(P_res), Switch/2, Droop Batt/5("Psource ")
  [P_RES] -> First-Order Filter/1

== system PV_MG_DroopMPPTV4_TwoFarms/Control /Current Controller ==
  I_measured : Inport  SampleTime=5e-5
  I_ref : Inport  Port=2  SampleTime=5e-5
  delata_I : Inport  Port=3
  Abs : Abs
  Fuzzy Control : Subsystem  TreatAsAtomicUnit=on
  Hysteric Control : Subsystem  TreatAsAtomicUnit=on
  If : If  IfExpression=u1 < 30
  Merge : Merge
  Sum2 : Sum  Inputs=|+-
  G : Outport
  wires:
  If/1 -> Hysteric Control/Action
  If/2 -> Fuzzy Control/Action
  I_ref/1 -> Sum2/1, Hysteric Control/1(I_ref), Fuzzy Control/1(I_ref)
  I_measured/1 -> Hysteric Control/3(I_measured), Fuzzy Control/2(I_measured), Sum2/2
  Fuzzy Control/1(G) -> Merge/2
  delata_I/1 -> Hysteric Control/2(delta_I)
  Hysteric Control/1(G) -> Merge/1
  Sum2/1 -> Abs/1
  Abs/1 -> If/1
  Merge/1 -> G/1

== system PV_MG_DroopMPPTV4_TwoFarms/Control /Current Controller1 ==
  I_measured : Inport  SampleTime=5e-5
  I_ref : Inport  Port=2  SampleTime=5e-5
  delata_I : Inport  Port=3
  Abs : Abs
  Fuzzy Control : Subsystem  TreatAsAtomicUnit=on
  Hysteric Control : Subsystem  TreatAsAtomicUnit=on
  If : If  IfExpression=u1 < 30
  Merge : Merge
  Sum2 : Sum  Inputs=|+-
  G : Outport
  wires:
  Merge/1 -> G/1
  Abs/1 -> If/1
  Sum2/1 -> Abs/1
  Hysteric Control/1(G) -> Merge/1
  delata_I/1 -> Hysteric Control/2(delta_I)
  Fuzzy Control/1(G) -> Merge/2
  I_measured/1 -> Sum2/2, Fuzzy Control/2(I_measured), Hysteric Control/3(I_measured)
  I_ref/1 -> Fuzzy Control/1(I_ref), Hysteric Control/1(I_ref), Sum2/1
  If/2 -> Fuzzy Control/Action
  If/1 -> Hysteric Control/Action

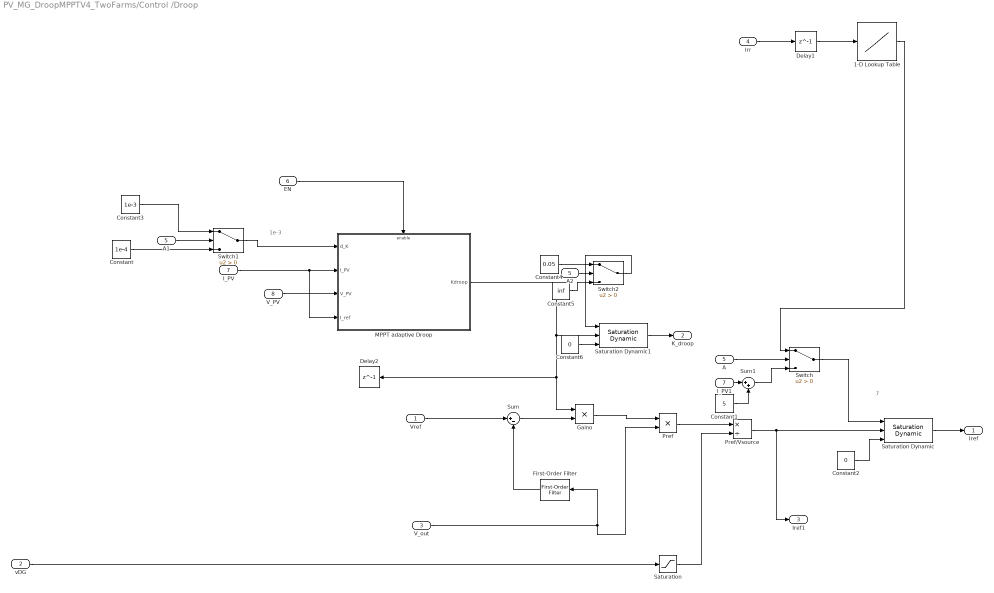
== system PV_MG_DroopMPPTV4_TwoFarms/Control /Droop ==
  note: 1e-3
  note: 7
  Vref : Inport
  vDG : Inport  Port=2
  V_out : Inport  Port=3
  Irr : Inport  Port=4
  A : Inport  Port=5
  EN : Inport  Port=6
  I_PV : Inport  Port=7
  V_PV : Inport  Port=8
  1-D Lookup Table : Lookup_n-D  NumberOfTableDimensions=1  BreakpointsForDimension1=fliplr([1000 900 800 600 500 400 300 200 100 0])  Table=fliplr([17 16.5 15 14.5 11 8 2.5 2 1.5 0])  InternalRulePriority=Speed  RndMeth=Simplest  InputSameDT=on
  A1 : InportShadow  Port=5
  A2 : InportShadow  Port=5
  Constant : Constant  Value=1e-4
  Constant1 : Constant  Value=5  SampleTime=0
  Constant2 : Constant  Value=0  SampleTime=0
  Constant3 : Constant  Value=1e-3
  Constant4 : Constant  Value=0.05  SampleTime=0
  Constant5 : Constant  Value=inf  SampleTime=0
  Constant6 : Constant  Value=0  SampleTime=0
  Delay1 : Delay  DelayLength=1  InitialCondition=0
  Delay2 : Delay  DelayLength=1  InitialCondition=0
  First-Order Filter : powerlib_meascontrol/Filters/First-Order Filter  FilterType=Lowpass  Tc=1/8000  Ts=0  Initialize=off  Vac_Init=[0, 0, 60]  Vdc_Init=0  PlotResponse=off  FreqRange="[0,  5000,  1]"
  Gaino : Product
  I_PV1 : InportShadow  Port=7
  MPPT adaptive Droop : Subsystem  TreatAsAtomicUnit=on
  Pref : Product
  Pref/Vsource : Product  Inputs=*/
  Saturation : Saturate  UpperLimit=inf  LowerLimit=1
  Saturation Dynamic : simulink/Discontinuities/Saturation Dynamic  OutMin=[]  OutMax=[]  OutDataTypeStr=Inherit: Same as second input  OutDataType=fixdt(1, 16)  OutScaling=2^-10  DoSatur=off
  Saturation Dynamic1 : simulink/Discontinuities/Saturation Dynamic  OutMin=[]  OutMax=[]  OutDataTypeStr=Inherit: Same as second input  OutDataType=fixdt(1, 16)  OutScaling=2^-10  DoSatur=off
  Sum : Sum  Inputs=|+-
  Sum1 : Sum  Inputs=|++
  Switch : Switch  Criteria=u2 > Threshold
  Switch1 : Switch  Criteria=u2 > Threshold
  Switch2 : Switch  Criteria=u2 > Threshold
  Iref : Outport
  K_droop : Outport  Port=2
  Iref1 : Outport  Port=3
  wires:
  Sum/1 -> Gaino/2
  First-Order Filter/1 -> Sum/2
  Pref/1 -> Pref/Vsource/1
  Saturation/1 -> Pref/Vsource/2
  Gaino/1 -> Pref/1
  Pref/Vsource/1 -> Saturation Dynamic/2, Iref1/1
  V_out/1 -> Pref/2, First-Order Filter/1
  Vref/1 -> Sum/1
  Constant2/1 -> Saturation Dynamic/3
  Delay1/1 -> 1-D Lookup Table/1
  Irr/1 -> Delay1/1
  Saturation Dynamic/1 -> Iref/1
  Switch/1 -> Saturation Dynamic/1
  1-D Lookup Table/1 -> Switch/1
  Sum1/1 -> Switch/3
  A/1 -> Switch/2
  Constant/1 -> Switch1/3
  A1/1 -> Switch1/2
  Constant3/1 -> Switch1/1
  Switch1/1 -> MPPT adaptive Droop/1(d_K)
  vDG/1 -> Saturation/1
  EN/1 -> MPPT adaptive Droop/Enable
  V_PV/1 -> MPPT adaptive Droop/3(V_PV)
  I_PV/1 -> MPPT adaptive Droop/4(I_ref), MPPT adaptive Droop/2(I_PV)
  MPPT adaptive Droop/1(Kdroop) -> Saturation Dynamic1/2, Delay2/1, Gaino/1
  Saturation Dynamic1/1 -> K_droop/1
  Constant4/1 -> Switch2/1
  Switch2/1 -> Saturation Dynamic1/1
  Constant5/1 -> Switch2/3
  A2/1 -> Switch2/2
  Constant6/1 -> Saturation Dynamic1/3
  I_PV1/1 -> Sum1/1
  Constant1/1 -> Sum1/2

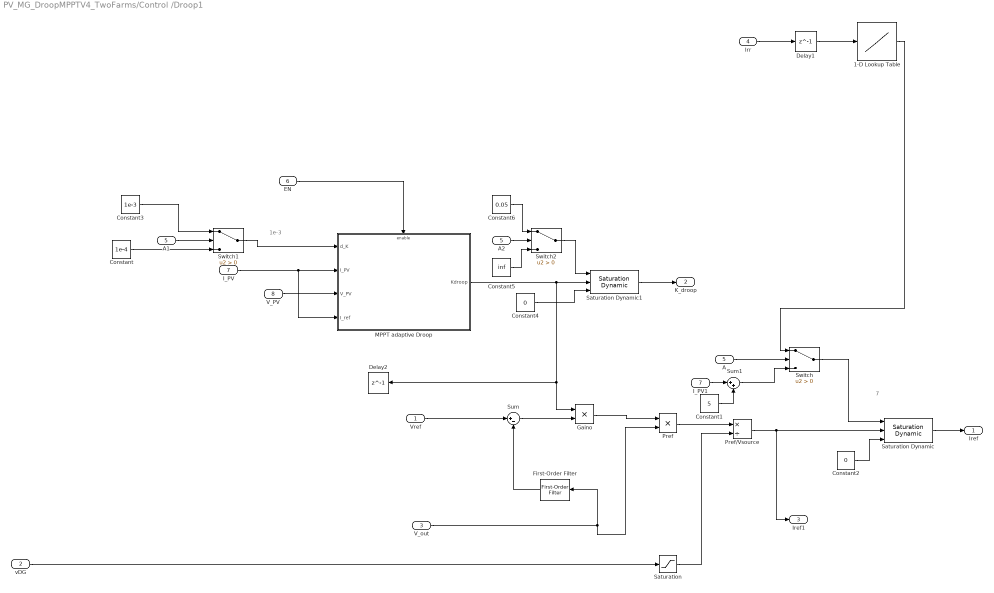
== system PV_MG_DroopMPPTV4_TwoFarms/Control /Droop1 ==
  note: 7
  note: 1e-3
  Vref : Inport
  vDG : Inport  Port=2
  V_out : Inport  Port=3
  Irr : Inport  Port=4
  A : Inport  Port=5
  EN : Inport  Port=6
  I_PV : Inport  Port=7
  V_PV : Inport  Port=8
  1-D Lookup Table : Lookup_n-D  NumberOfTableDimensions=1  BreakpointsForDimension1=fliplr([1000 900 800 600 500 400 300 200 100 0])  Table=fliplr([17 16.5 15 14.5 11 8 2.5 2 1.5 0])  InternalRulePriority=Speed  RndMeth=Simplest  InputSameDT=on
  A1 : InportShadow  Port=5
  A2 : InportShadow  Port=5
  Constant : Constant  Value=1e-4
  Constant1 : Constant  Value=5  SampleTime=0
  Constant2 : Constant  Value=0  SampleTime=0
  Constant3 : Constant  Value=1e-3
  Constant4 : Constant  Value=0  SampleTime=0
  Constant5 : Constant  Value=inf  SampleTime=0
  Constant6 : Constant  Value=0.05  SampleTime=0
  Delay1 : Delay  DelayLength=1  InitialCondition=0
  Delay2 : Delay  DelayLength=1  InitialCondition=0
  First-Order Filter : powerlib_meascontrol/Filters/First-Order Filter  FilterType=Lowpass  Tc=1/8000  Ts=0  Initialize=off  Vac_Init=[0, 0, 60]  Vdc_Init=0  PlotResponse=off  FreqRange="[0,  5000,  1]"
  Gaino : Product
  I_PV1 : InportShadow  Port=7
  MPPT adaptive Droop : Subsystem  TreatAsAtomicUnit=on
  Pref : Product
  Pref/Vsource : Product  Inputs=*/
  Saturation : Saturate  UpperLimit=inf  LowerLimit=1
  Saturation Dynamic : simulink/Discontinuities/Saturation Dynamic  OutMin=[]  OutMax=[]  OutDataTypeStr=Inherit: Same as second input  OutDataType=fixdt(1, 16)  OutScaling=2^-10  DoSatur=off
  Saturation Dynamic1 : simulink/Discontinuities/Saturation Dynamic  OutMin=[]  OutMax=[]  OutDataTypeStr=Inherit: Same as second input  OutDataType=fixdt(1, 16)  OutScaling=2^-10  DoSatur=off
  Sum : Sum  Inputs=|+-
  Sum1 : Sum  Inputs=|++
  Switch : Switch  Criteria=u2 > Threshold
  Switch1 : Switch  Criteria=u2 > Threshold
  Switch2 : Switch  Criteria=u2 > Threshold
  Iref : Outport
  K_droop : Outport  Port=2
  Iref1 : Outport  Port=3
  wires:
  MPPT adaptive Droop/1(Kdroop) -> Saturation Dynamic1/2, Gaino/1, Delay2/1
  I_PV/1 -> MPPT adaptive Droop/4(I_ref), MPPT adaptive Droop/2(I_PV)
  V_PV/1 -> MPPT adaptive Droop/3(V_PV)
  EN/1 -> MPPT adaptive Droop/Enable
  vDG/1 -> Saturation/1
  Switch1/1 -> MPPT adaptive Droop/1(d_K)
  Constant3/1 -> Switch1/1
  A1/1 -> Switch1/2
  Constant/1 -> Switch1/3
  A/1 -> Switch/2
  Sum1/1 -> Switch/3
  1-D Lookup Table/1 -> Switch/1
  Switch/1 -> Saturation Dynamic/1
  Saturation Dynamic/1 -> Iref/1
  Irr/1 -> Delay1/1
  Delay1/1 -> 1-D Lookup Table/1
  Constant2/1 -> Saturation Dynamic/3
  Vref/1 -> Sum/1
  V_out/1 -> First-Order Filter/1, Pref/2
  Pref/Vsource/1 -> Iref1/1, Saturation Dynamic/2
  Gaino/1 -> Pref/1
  Saturation/1 -> Pref/Vsource/2
  Pref/1 -> Pref/Vsource/1
  First-Order Filter/1 -> Sum/2
  Sum/1 -> Gaino/2
  Saturation Dynamic1/1 -> K_droop/1
  Switch2/1 -> Saturation Dynamic1/1
  A2/1 -> Switch2/2
  Constant4/1 -> Saturation Dynamic1/3
  Constant5/1 -> Switch2/3
  Constant6/1 -> Switch2/1
  I_PV1/1 -> Sum1/1
  Constant1/1 -> Sum1/2

== system PV_MG_DroopMPPTV4_TwoFarms/Monitor And Input/Lamp3 ==

== system PV_MG_DroopMPPTV4_TwoFarms/Monitor And Input/Rocker Switch1 ==

== system PV_MG_DroopMPPTV4_TwoFarms/Monitor And Input/Rocker Switch2 ==

== system PV_MG_DroopMPPTV4_TwoFarms/Control /Battery Control/Bi-Current Controller ==
  I_ref : Inport  SampleTime=5e-5
  I_discharge : Inport  Port=2  SampleTime=5e-5
  I_charge : Inport  Port=3  SampleTime=5e-5
  delta_I : Inport  Port=4
  Abs : Abs
  Abs1 : Abs
  Fuzzy Control : Subsystem  TreatAsAtomicUnit=on
  Hysteric Control : Subsystem  TreatAsAtomicUnit=on
  If : If  IfExpression=u1 < 30
  Merge : Merge
  Merge1 : Merge
  Merge2 : Merge
  Sum2 : Sum  Inputs=|+-
  Switch : Switch  Criteria=u2 > Threshold
  G : Outport
  Light : Outport  Port=2
  Duty : Outport  Port=3
  wires:
  If/1 -> Hysteric Control/Action
  If/2 -> Fuzzy Control/Action
  Fuzzy Control/1(G) -> Merge/2
  Hysteric Control/1(G) -> Merge/1
  Hysteric Control/2(Lamp) -> Merge1/1
  Fuzzy Control/2(lamp) -> Merge1/2
  Sum2/1 -> Abs/1
  Abs/1 -> If/1
  Fuzzy Control/3(D1) -> Merge2/2
  Hysteric Control/3(D1) -> Merge2/1
  Merge/1 -> G/1
  Merge2/1 -> Duty/1
  Merge1/1 -> Light/1
  Switch/1 -> Fuzzy Control/2(I_measured), Hysteric Control/3(I_measured), Sum2/2
  delta_I/1 -> Hysteric Control/2(delta_I)
  I_discharge/1 -> Switch/1
  I_charge/1 -> Switch/3
  I_ref/1 -> Abs1/1, Switch/2
  Abs1/1 -> Sum2/1, Hysteric Control/1(I_ref), Fuzzy Control/1(I_ref)

== system PV_MG_DroopMPPTV4_TwoFarms/Control /Battery Control/Droop Batt ==
  Vref : Inport
  vDG : Inport  Port=2
  I_L : Inport  Port=3
  V_out : Inport  Port=4
  "Psource " : Inport  Port=5
  Constant : Constant  Value=0.15  SampleTime=0
  Constant1 : Constant  SampleTime=0
  Enabled Subsystem : Subsystem  TreatAsAtomicUnit=on
  First-Order Filter : powerlib_meascontrol/Filters/First-Order Filter  FilterType=Lowpass  Tc=1/8000  Ts=0  Initialize=off  Vac_Init=[0, 0, 60]  Vdc_Init=0  PlotResponse=off  FreqRange="[0,  5000,  1]"
  Gaino : Product
  Pref : Product
  Pref/Vsource : Product  Inputs=*/
  Saturation : Saturate  UpperLimit=inf  LowerLimit=0.000001
  Saturation1 : Saturate  UpperLimit=100  LowerLimit=0
  Sum : Sum  Inputs=|+-
  Switch : Switch  Criteria=u2 ~= 0
  Iref : Outport
  K_droop : Outport  Port=2
  wires:
  Constant1/1 -> Switch/2
  Switch/1 -> Gaino/1, K_droop/1
  Constant/1 -> Switch/3
  Enabled Subsystem/1(Kdroop) -> Switch/1
  Saturation1/1 -> Iref/1
  "Psource "/1 -> Enabled Subsystem/3(Psource)
  I_L/1 -> Enabled Subsystem/1(I_l)
  V_out/1 -> Pref/2, First-Order Filter/1
  Pref/Vsource/1 -> Saturation1/1
  Gaino/1 -> Pref/1
  vDG/1 -> Saturation/1, Enabled Subsystem/2(V_G)
  Vref/1 -> Sum/1
  Saturation/1 -> Pref/Vsource/2
  Pref/1 -> Pref/Vsource/1
  First-Order Filter/1 -> Sum/2
  Sum/1 -> Gaino/2

== system PV_MG_DroopMPPTV4_TwoFarms/Control /Battery Control/Subsystem ==
  V_Batt : Inport
  P_res : Inport  Port=2
  Divide : Product  Inputs=*/
  I_ref : Outport
  wires:
  P_res/1 -> Divide/1
  V_Batt/1 -> Divide/2
  Divide/1 -> I_ref/1

== system PV_MG_DroopMPPTV4_TwoFarms/Control /Current Controller/Fuzzy Control ==
  note: Filterout oscillations due to switching frequency
  I_ref : Inport
  I_measured : Inport  Port=2
  Action Port : ActionPort  ActionType=else
  Discrete Filter1 : DiscreteFilter  Numerator=[1 -1]  Denominator=[1]
  First-Order Filter : powerlib_meascontrol/Filters/First-Order Filter  FilterType=Lowpass  Tc=1/8000  Ts=5e-5  Initialize=off  Vac_Init=[0, 0, 60]  Vdc_Init=0  PlotResponse=off  FreqRange="[0,  5000,  1]"
  Fuzzy Logic Controller : fuzblock/Fuzzy Logic  Controller  fis=ZIloop5
  Mux : Mux  Inputs=2
  PWM Generator (DC-DC) : powerlib_meascontrol/Pulse & Signal Generators/PWM Generator (DC-DC)  Fsw=10000  Ts=5e-5
  Saturation : Saturate  UpperLimit=0.8  LowerLimit=0
  Saturation1 : Saturate  UpperLimit=100  LowerLimit=-100
  Saturation2 : Saturate  UpperLimit=10  LowerLimit=-10
  Sum : Sum  Inputs=|+-
  G : Outport
  wires:
  Mux/1 -> Fuzzy Logic Controller/1
  I_ref/1 -> Sum/1
  Saturation/1 -> PWM Generator (DC-DC)/1
  PWM Generator (DC-DC)/1 -> G/1
  Sum/1 -> Saturation1/1
  Saturation1/1 -> Mux/1, Discrete Filter1/1
  Discrete Filter1/1 -> Saturation2/1
  Saturation2/1 -> Mux/2
  I_measured/1 -> First-Order Filter/1
  First-Order Filter/1 -> Sum/2
  Fuzzy Logic Controller/1 -> Saturation/1

== system PV_MG_DroopMPPTV4_TwoFarms/Control /Current Controller/Hysteric Control ==
  I_ref : Inport
  delta_I : Inport  Port=2
  I_measured : Inport  Port=3
  Action Port : ActionPort  ActionType=then
  Data Type Conversion : DataTypeConversion  OutDataTypeStr=boolean
  Data Type Conversion1 : DataTypeConversion  OutDataTypeStr=boolean
  Data Type Conversion2 : DataTypeConversion  OutDataTypeStr=double
  Relational Operator : RelationalOperator  OutDataTypeStr=boolean  ZeroCross=off
  Relational Operator1 : RelationalOperator  Operator=<=  OutDataTypeStr=boolean  ZeroCross=off
  S-R Flip-Flop : simulink_extras/Flip Flops/S-R Flip-Flop  initial_condition=0
  Saturation : Saturate  UpperLimit=1  LowerLimit=0
  Sum : Sum  Inputs=|+-
  Sum1 : Sum  Inputs=|++
  G : Outport
  wires:
  I_ref/1 -> Sum1/1, Sum/1
  delta_I/1 -> Sum/2, Sum1/2
  Data Type Conversion/1 -> S-R Flip-Flop/1
  Data Type Conversion1/1 -> S-R Flip-Flop/2
  Sum/1 -> Relational Operator/1
  Relational Operator/1 -> Data Type Conversion/1
  Relational Operator1/1 -> Data Type Conversion1/1
  Sum1/1 -> Relational Operator1/1
  I_measured/1 -> Relational Operator/2, Relational Operator1/2
  Data Type Conversion2/1 -> Saturation/1
  Saturation/1 -> G/1
  S-R Flip-Flop/1 -> Data Type Conversion2/1

== system PV_MG_DroopMPPTV4_TwoFarms/Control /Current Controller1/Fuzzy Control ==
  note: Filterout oscillations due to switching frequency
  I_ref : Inport
  I_measured : Inport  Port=2
  Action Port : ActionPort  ActionType=else
  Discrete Filter1 : DiscreteFilter  Numerator=[1 -1]  Denominator=[1]
  First-Order Filter : powerlib_meascontrol/Filters/First-Order Filter  FilterType=Lowpass  Tc=1/8000  Ts=5e-5  Initialize=off  Vac_Init=[0, 0, 60]  Vdc_Init=0  PlotResponse=off  FreqRange="[0,  5000,  1]"
  Fuzzy Logic Controller : fuzblock/Fuzzy Logic  Controller  fis=ZIloop5
  Mux : Mux  Inputs=2
  PWM Generator (DC-DC) : powerlib_meascontrol/Pulse & Signal Generators/PWM Generator (DC-DC)  Fsw=10000  Ts=5e-5
  Saturation : Saturate  UpperLimit=0.8  LowerLimit=0
  Saturation1 : Saturate  UpperLimit=100  LowerLimit=-100
  Saturation2 : Saturate  UpperLimit=10  LowerLimit=-10
  Sum : Sum  Inputs=|+-
  G : Outport
  wires:
  Fuzzy Logic Controller/1 -> Saturation/1
  First-Order Filter/1 -> Sum/2
  I_measured/1 -> First-Order Filter/1
  Saturation2/1 -> Mux/2
  Discrete Filter1/1 -> Saturation2/1
  Saturation1/1 -> Discrete Filter1/1, Mux/1
  Sum/1 -> Saturation1/1
  PWM Generator (DC-DC)/1 -> G/1
  Saturation/1 -> PWM Generator (DC-DC)/1
  I_ref/1 -> Sum/1
  Mux/1 -> Fuzzy Logic Controller/1

== system PV_MG_DroopMPPTV4_TwoFarms/Control /Current Controller1/Hysteric Control ==
  I_ref : Inport
  delta_I : Inport  Port=2
  I_measured : Inport  Port=3
  Action Port : ActionPort  ActionType=then
  Data Type Conversion : DataTypeConversion  OutDataTypeStr=boolean
  Data Type Conversion1 : DataTypeConversion  OutDataTypeStr=boolean
  Data Type Conversion2 : DataTypeConversion  OutDataTypeStr=double
  Relational Operator : RelationalOperator  OutDataTypeStr=boolean  ZeroCross=off
  Relational Operator1 : RelationalOperator  Operator=<=  OutDataTypeStr=boolean  ZeroCross=off
  S-R Flip-Flop : simulink_extras/Flip Flops/S-R Flip-Flop  initial_condition=0
  Saturation : Saturate  UpperLimit=1  LowerLimit=0
  Sum : Sum  Inputs=|+-
  Sum1 : Sum  Inputs=|++
  G : Outport
  wires:
  S-R Flip-Flop/1 -> Data Type Conversion2/1
  Saturation/1 -> G/1
  Data Type Conversion2/1 -> Saturation/1
  I_measured/1 -> Relational Operator1/2, Relational Operator/2
  Sum1/1 -> Relational Operator1/1
  Relational Operator1/1 -> Data Type Conversion1/1
  Relational Operator/1 -> Data Type Conversion/1
  Sum/1 -> Relational Operator/1
  Data Type Conversion1/1 -> S-R Flip-Flop/2
  Data Type Conversion/1 -> S-R Flip-Flop/1
  delta_I/1 -> Sum1/2, Sum/2
  I_ref/1 -> Sum/1, Sum1/1

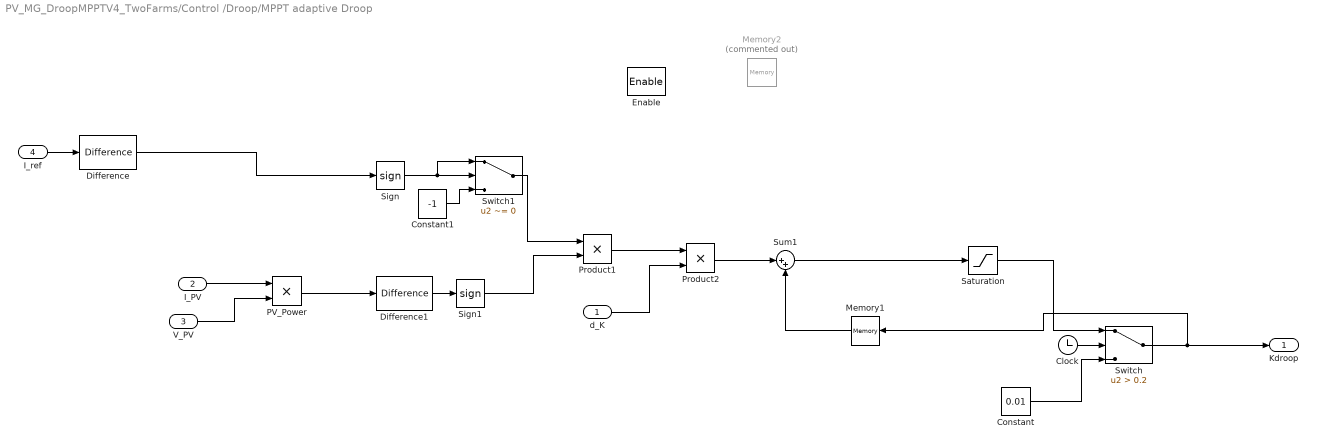
== system PV_MG_DroopMPPTV4_TwoFarms/Control /Droop/MPPT adaptive Droop ==
  d_K : Inport
  I_PV : Inport  Port=2
  V_PV : Inport  Port=3
  I_ref : Inport  Port=4
  Enable : EnablePort
  Clock : Clock
  Constant : Constant  Value=0.01
  Constant1 : Constant  Value=-1
  Difference : simulink/Discrete/Difference  ICPrevInput=0.0  InputProcessing=Inherited  OutMin=[]  OutMax=[]  OutDataType=fixdt(1, 16)  OutScaling=2^-10  DoSatur=off
  Difference1 : simulink/Discrete/Difference  ICPrevInput=0.0  InputProcessing=Inherited  OutMin=[]  OutMax=[]  OutDataType=fixdt(1, 16)  OutScaling=2^-10  DoSatur=off
  Memory1 : Memory
  Memory2 : Memory  Commented=on
  PV_Power : Product
  Product1 : Product
  Product2 : Product
  Saturation : Saturate  UpperLimit=4  LowerLimit=0
  Sign : Signum
  Sign1 : Signum
  Sum1 : Sum  Inputs=|++
  Switch : Switch  Criteria=u2 > Threshold  Threshold=0.2
  Switch1 : Switch  Criteria=u2 ~= 0  Threshold=0.1
  Kdroop : Outport
  wires:
  PV_Power/1 -> Difference1/1
  Difference1/1 -> Sign1/1
  Sign1/1 -> Product1/2
  Product1/1 -> Product2/1
  d_K/1 -> Product2/2
  Product2/1 -> Sum1/1
  Memory1/1 -> Sum1/2
  Sum1/1 -> Saturation/1
  Constant/1 -> Switch/3
  Switch/1 -> Kdroop/1, Memory1/1
  Saturation/1 -> Switch/1
  Sign/1 -> Switch1/1, Switch1/2
  Constant1/1 -> Switch1/3
  Switch1/1 -> Product1/1
  Difference/1 -> Sign/1
  I_PV/1 -> PV_Power/1
  V_PV/1 -> PV_Power/2
  I_ref/1 -> Difference/1
  Clock/1 -> Switch/2

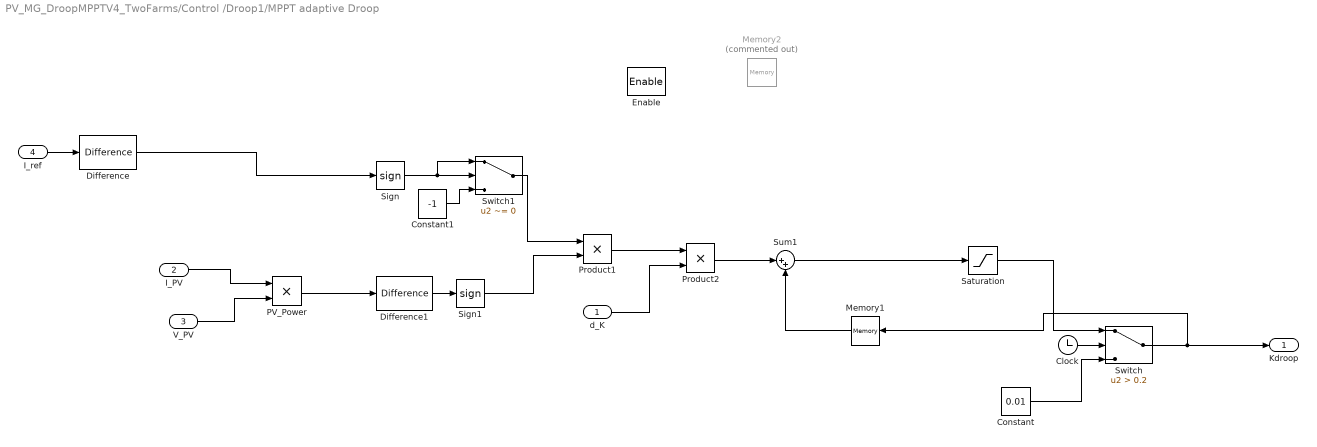
== system PV_MG_DroopMPPTV4_TwoFarms/Control /Droop1/MPPT adaptive Droop ==
  d_K : Inport
  I_PV : Inport  Port=2
  V_PV : Inport  Port=3
  I_ref : Inport  Port=4
  Enable : EnablePort
  Clock : Clock
  Constant : Constant  Value=0.01
  Constant1 : Constant  Value=-1
  Difference : simulink/Discrete/Difference  ICPrevInput=0.0  InputProcessing=Inherited  OutMin=[]  OutMax=[]  OutDataType=fixdt(1, 16)  OutScaling=2^-10  DoSatur=off
  Difference1 : simulink/Discrete/Difference  ICPrevInput=0.0  InputProcessing=Inherited  OutMin=[]  OutMax=[]  OutDataType=fixdt(1, 16)  OutScaling=2^-10  DoSatur=off
  Memory1 : Memory
  Memory2 : Memory  Commented=on
  PV_Power : Product
  Product1 : Product
  Product2 : Product
  Saturation : Saturate  UpperLimit=4  LowerLimit=0
  Sign : Signum
  Sign1 : Signum
  Sum1 : Sum  Inputs=|++
  Switch : Switch  Criteria=u2 > Threshold  Threshold=0.2
  Switch1 : Switch  Criteria=u2 ~= 0  Threshold=0.1
  Kdroop : Outport
  wires:
  Clock/1 -> Switch/2
  I_ref/1 -> Difference/1
  V_PV/1 -> PV_Power/2
  I_PV/1 -> PV_Power/1
  Difference/1 -> Sign/1
  Switch1/1 -> Product1/1
  Constant1/1 -> Switch1/3
  Sign/1 -> Switch1/2, Switch1/1
  Saturation/1 -> Switch/1
  Switch/1 -> Memory1/1, Kdroop/1
  Constant/1 -> Switch/3
  Sum1/1 -> Saturation/1
  Memory1/1 -> Sum1/2
  Product2/1 -> Sum1/1
  d_K/1 -> Product2/2
  Product1/1 -> Product2/1
  Sign1/1 -> Product1/2
  Difference1/1 -> Sign1/1
  PV_Power/1 -> Difference1/1
